simulink model "Nonlinear_System_Stability_Design"  (R2020b)
settings: Solver=VariableStepAuto  StartTime=0.0  StopTime=10.0  RelTol=1e-3
undefined symbols (not defined in the file): magnitude
settings Model: Creator=24365  LastModifiedBy=24365

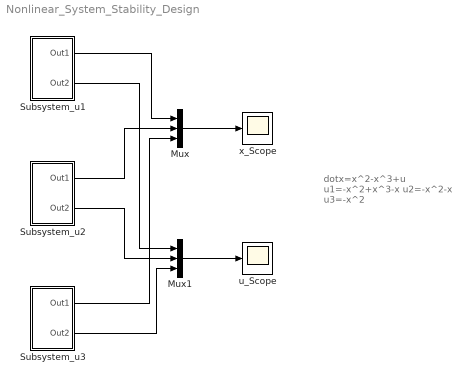
== system Nonlinear_System_Stability_Design ==
  note: dotx=x^2-x^3+u
      | u1=-x^2+x^3-x
      | u2=-x^2-x
      | u3=-x^2
  Mux : Mux  Inputs=3
  Mux1 : Mux  Inputs=3
  Subsystem_u1 : Subsystem
  Subsystem_u2 : Subsystem
  Subsystem_u3 : Subsystem
  u_Scope : Scope
  x_Scope : Scope
  wires:
  Subsystem_u1/1(Out1) -> Mux/1
  Mux/1 -> x_Scope/1
  Subsystem_u1/2(Out2) -> Mux1/1
  Mux1/1 -> u_Scope/1
  Subsystem_u2/1(Out1) -> Mux/2
  Subsystem_u2/2(Out2) -> Mux1/2
  Subsystem_u3/1(Out1) -> Mux/3
  Subsystem_u3/2(Out2) -> Mux1/3

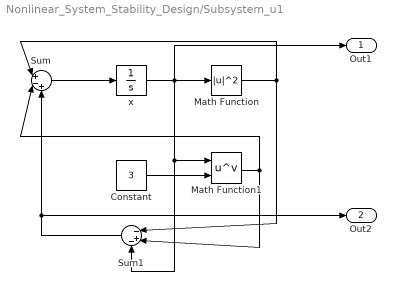
== system Nonlinear_System_Stability_Design/Subsystem_u1 ==
  Constant : Constant  Value=3
  Math Function : Math  Operator=magnitude^2  SaturateOnIntegerOverflow=on
  Math Function1 : Math  Operator=pow  SaturateOnIntegerOverflow=on
  Sum : Sum  Inputs=|+-+
  Sum1 : Sum  Inputs=|-+-
  x : Integrator  InitialCondition=10
  Out1 : Outport
  Out2 : Outport  Port=2
  wires:
  Math Function/1 -> Sum1/1, Sum/1
  x/1 -> Out1/1, Sum1/3, Math Function1/1, Math Function/1
  Math Function1/1 -> Sum1/2, Sum/2
  Sum/1 -> x/1
  Constant/1 -> Math Function1/2
  Sum1/1 -> Out2/1, Sum/3

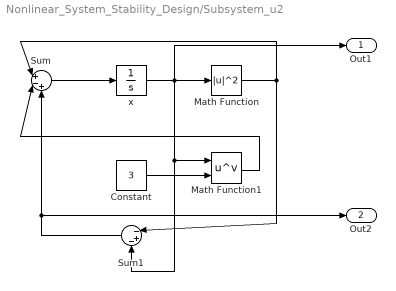
== system Nonlinear_System_Stability_Design/Subsystem_u2 ==
  Constant : Constant  Value=3
  Math Function : Math  Operator=magnitude^2  SaturateOnIntegerOverflow=on
  Math Function1 : Math  Operator=pow  SaturateOnIntegerOverflow=on
  Sum : Sum  Inputs=|+-+
  Sum1 : Sum  Inputs=|-+-
  x : Integrator  InitialCondition=10
  Out1 : Outport
  Out2 : Outport  Port=2
  wires:
  Sum1/1 -> Sum/3, Out2/1
  Constant/1 -> Math Function1/2
  Sum/1 -> x/1
  Math Function1/1 -> Sum/2
  x/1 -> Math Function/1, Math Function1/1, Sum1/3, Out1/1
  Math Function/1 -> Sum/1, Sum1/1

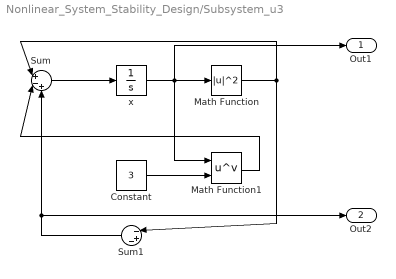
== system Nonlinear_System_Stability_Design/Subsystem_u3 ==
  Constant : Constant  Value=3
  Math Function : Math  Operator=magnitude^2  SaturateOnIntegerOverflow=on
  Math Function1 : Math  Operator=pow  SaturateOnIntegerOverflow=on
  Sum : Sum  Inputs=|+-+
  Sum1 : Sum  Inputs=|-+-
  x : Integrator  InitialCondition=10
  Out1 : Outport
  Out2 : Outport  Port=2
  wires:
  Math Function/1 -> Sum1/1, Sum/1
  x/1 -> Out1/1, Math Function1/1, Math Function/1
  Math Function1/1 -> Sum/2
  Sum/1 -> x/1
  Constant/1 -> Math Function1/2
  Sum1/1 -> Out2/1, Sum/3
